simulink subsystem "pulse_logic"  (R2021a)
settings: Solver=VariableStepAuto  StartTime=0.0  StopTime=10.0  RelTol=1e-3
libraries: xbsIndex_r4 x101
settings Model: Creator=casper  LastModifiedBy=casper

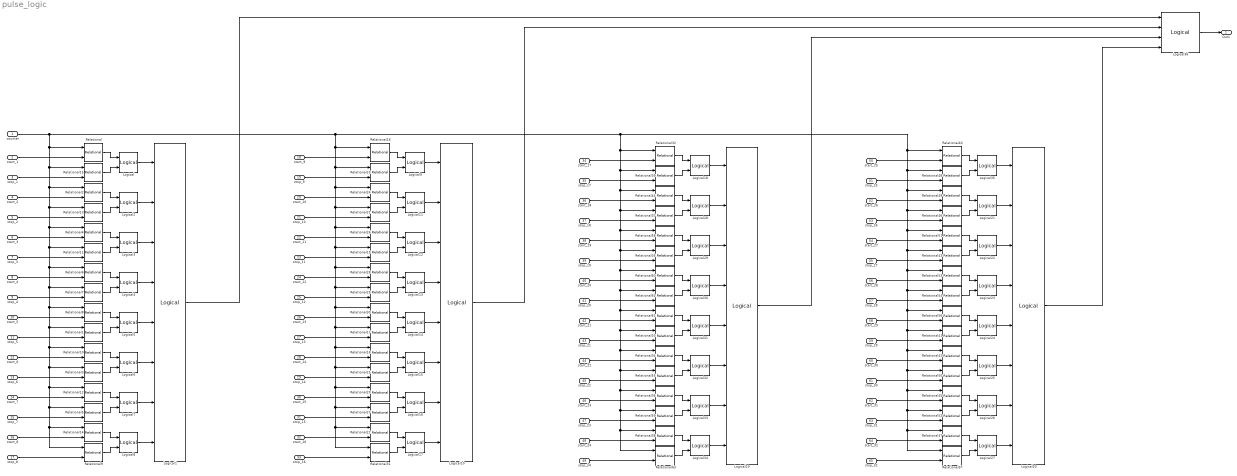
== system pulse_logic ==
  counter : Inport
  start_1 : Inport  Port=2
  stop_1 : Inport  Port=3
  start_2 : Inport  Port=4
  stop_2 : Inport  Port=5
  start_3 : Inport  Port=6
  stop_3 : Inport  Port=7
  start_4 : Inport  Port=8
  stop_4 : Inport  Port=9
  start_5 : Inport  Port=10
  stop_5 : Inport  Port=11
  start_6 : Inport  Port=12
  stop_6 : Inport  Port=13
  start_7 : Inport  Port=14
  stop_7 : Inport  Port=15
  start_8 : Inport  Port=16
  stop_8 : Inport  Port=17
  start_9 : Inport  Port=18
  stop_9 : Inport  Port=19
  start_10 : Inport  Port=20
  stop_10 : Inport  Port=21
  start_11 : Inport  Port=22
  stop_11 : Inport  Port=23
  start_12 : Inport  Port=24
  stop_12 : Inport  Port=25
  start_13 : Inport  Port=26
  stop_13 : Inport  Port=27
  start_14 : Inport  Port=28
  stop_14 : Inport  Port=29
  start_15 : Inport  Port=30
  stop_15 : Inport  Port=31
  start_16 : Inport  Port=32
  stop_16 : Inport  Port=33
  start_17 : Inport  Port=34
  stop_17 : Inport  Port=35
  start_18 : Inport  Port=36
  stop_18 : Inport  Port=37
  start_19 : Inport  Port=38
  stop_19 : Inport  Port=39
  start_20 : Inport  Port=40
  stop_20 : Inport  Port=41
  start_21 : Inport  Port=42
  stop_21 : Inport  Port=43
  start_22 : Inport  Port=44
  stop_22 : Inport  Port=45
  start_23 : Inport  Port=46
  stop_23 : Inport  Port=47
  start_24 : Inport  Port=48
  stop_24 : Inport  Port=49
  start_25 : Inport  Port=50
  stop_25 : Inport  Port=51
  start_26 : Inport  Port=52
  stop_26 : Inport  Port=53
  start_27 : Inport  Port=54
  stop_27 : Inport  Port=55
  start_28 : Inport  Port=56
  stop_28 : Inport  Port=57
  start_29 : Inport  Port=58
  stop_29 : Inport  Port=59
  start_30 : Inport  Port=60
  stop_30 : Inport  Port=61
  start_31 : Inport  Port=62
  stop_31 : Inport  Port=63
  start_32 : Inport  Port=64
  stop_32 : Inport  Port=65
  Logical{,2..9,11..18,21..35} (32 alike) : xbsIndex_r4/Logical  logical_function=AND  inputs=2  en=off  latency=1  precision=Full  arith_type=Unsigned  n_bits=16  bin_pt=0  align_bp=on  dbl_ovrd=off  block_type=logical
  Logical{1,10,19..20} (4 alike) : xbsIndex_r4/Logical  logical_function=OR  inputs=8  en=off  latency=1  precision=Full  arith_type=Unsigned  n_bits=16  bin_pt=0  align_bp=on  dbl_ovrd=off  block_type=logical
  Logical36 : xbsIndex_r4/Logical  logical_function=OR  inputs=4  en=off  latency=1  precision=Full  arith_type=Unsigned  n_bits=16  bin_pt=0  align_bp=on  dbl_ovrd=off  block_type=logical
  Relational{,2,4,6,8,10,12,14,16,18,20,22,24,26,28,30,32,34,36,38,40,42,44..45,47,49,51,53,56,58,60,62} (32 alike) : xbsIndex_r4/Relational  mode=a>=b  op_type=Bool  en=off  latency=1  dbl_ovrd=off  block_type=relational
  Relational{1,3,5,7,9,11,13,15,17,19,21,23,25,27,29,31,33,35,37,39,41,43,46,48,50,52,54..55,57,59,61,63} (32 alike) : xbsIndex_r4/Relational  mode=a<b  op_type=Bool  en=off  latency=1  dbl_ovrd=off  block_type=relational
  Out1 : Outport
  wires:
  Logical5/1 -> Logical1/5
  Relational1/1 -> Logical5/2
  Relational9/1 -> Logical8/2
  Relational8/1 -> Logical5/1
  start_1/1 -> Relational/2
  Logical/1 -> Logical1/1
  stop_8/1 -> Relational9/2
  Relational2/1 -> Logical2/1
  Relational7/1 -> Logical4/2
  Relational6/1 -> Logical4/1
  Relational3/1 -> Logical6/2
  Logical4/1 -> Logical1/4
  start_5/1 -> Relational8/2
  Relational15/1 -> Logical/2
  Logical6/1 -> Logical1/6
  stop_6/1 -> Relational3/2
  stop_5/1 -> Relational1/2
  stop_7/1 -> Relational5/2
  Logical2/1 -> Logical1/2
  stop_1/1 -> Relational15/2
  start_4/1 -> Relational6/2
  stop_3/1 -> Relational11/2
  start_6/1 -> Relational10/2
  Relational4/1 -> Logical3/1
  start_3/1 -> Relational4/2
  Relational10/1 -> Logical6/1
  start_2/1 -> Relational2/2
  Relational/1 -> Logical/1
  stop_2/1 -> Relational13/2
  Logical8/1 -> Logical1/8
  Relational5/1 -> Logical7/2
  Relational11/1 -> Logical3/2
  Relational14/1 -> Logical8/1
  start_7/1 -> Relational12/2
  stop_4/1 -> Relational7/2
  start_8/1 -> Relational14/2
  Logical3/1 -> Logical1/3
  Relational12/1 -> Logical7/1
  Logical7/1 -> Logical1/7
  Relational13/1 -> Logical2/2
  Relational29/1 -> Logical13/2
  stop_12/1 -> Relational29/2
  stop_9/1 -> Relational23/2
  start_16/1 -> Relational22/2
  Logical11/1 -> Logical10/2
  stop_14/1 -> Relational25/2
  start_15/1 -> Relational20/2
  Logical15/1 -> Logical10/6
  Logical17/1 -> Logical10/8
  stop_10/1 -> Relational21/2
  Relational16/1 -> Logical9/1
  Relational24/1 -> Logical11/1
  Logical13/1 -> Logical10/4
  Relational25/1 -> Logical15/2
  Relational17/1 -> Logical14/2
  start_11/1 -> Relational26/2
  start_12/1 -> Relational28/2
  Logical12/1 -> Logical10/3
  Relational20/1 -> Logical16/1
  stop_16/1 -> Relational31/2
  Relational22/1 -> Logical17/1
  Relational27/1 -> Logical16/2
  Logical14/1 -> Logical10/5
  Relational26/1 -> Logical12/1
  start_10/1 -> Relational24/2
  Relational30/1 -> Logical14/1
  start_13/1 -> Relational30/2
  Relational28/1 -> Logical13/1
  Relational21/1 -> Logical11/2
  Relational19/1 -> Logical12/2
  stop_15/1 -> Relational27/2
  stop_13/1 -> Relational17/2
  start_14/1 -> Relational18/2
  Logical16/1 -> Logical10/7
  start_9/1 -> Relational16/2
  stop_11/1 -> Relational19/2
  Relational31/1 -> Logical17/2
  Relational23/1 -> Logical9/2
  Relational18/1 -> Logical15/1
  Logical9/1 -> Logical10/1
  stop_27/1 -> Relational43/2
  Logical26/1 -> Logical20/7
  start_30/1 -> Relational42/2
  stop_29/1 -> Relational41/2
  Relational43/1 -> Logical22/2
  Relational54/1 -> Logical23/2
  Relational33/1 -> Logical31/2
  start_26/1 -> Relational49/2
  Relational36/1 -> Logical33/1
  stop_23/1 -> Relational59/2
  stop_32/1 -> Relational57/2
  Relational41/1 -> Logical24/2
  Logical22/1 -> Logical20/3
  start_27/1 -> Relational51/2
  stop_28/1 -> Relational54/2
  start_18/1 -> Relational44/2
  Relational49/1 -> Logical21/1
  stop_30/1 -> Relational50/2
  Relational47/1 -> Logical27/1
  start_32/1 -> Relational47/2
  Relational53/1 -> Logical23/1
  Relational56/1 -> Logical24/1
  Relational51/1 -> Logical22/1
  Relational45/1 -> Logical26/1
  start_31/1 -> Relational45/2
  counter/1 -> Relational2/1, Relational13/1, Relational4/1, Relational11/1, Relational7/1, Relational8/1, Relational1/1, Relational10/1, Relational5/1, Relational14/1, Relational9/1, Relational12/1, Relational3/1, Relational6/1, Relational15/1, Relational/1, Relational24/1, Relational21/1, Relational26/1, Relational19/1, Relational29/1, Relational30/1, Relational17/1, Relational18/1, Relational27/1, Relational22/1, Relational31/1, Relational20/1, Relational25/1, Relational28/1, Relational23/1, Relational16/1, Relational44/1, Relational37/1, Relational58/1, Relational35/1, Relational61/1, Relational62/1, Relational33/1, Relational34/1, Relational59/1, Relational38/1, Relational63/1, Relational36/1, Relational55/1, Relational60/1, Relational39/1, Relational32/1, Relational49/1, Relational46/1, Relational51/1, Relational43/1, Relational54/1, Relational56/1, Relational41/1, Relational42/1, Relational52/1, Relational47/1, Relational57/1, Relational45/1, Relational50/1, Relational53/1, Relational48/1, Relational40/1
  stop_19/1 -> Relational35/2
  stop_25/1 -> Relational48/2
  stop_26/1 -> Relational46/2
  Logical27/1 -> Logical20/8
  Logical23/1 -> Logical20/4
  Logical25/1 -> Logical20/6
  Relational46/1 -> Logical21/2
  Logical33/1 -> Logical19/7
  start_17/1 -> Relational32/2
  start_29/1 -> Relational56/2
  Relational50/1 -> Logical25/2
  Logical29/1 -> Logical19/3
  Logical19/1 -> Logical36/3
  Logical18/1 -> Logical19/1
  Relational40/1 -> Logical35/1
  stop_21/1 -> Relational33/2
  Logical21/1 -> Logical20/2
  Relational48/1 -> Logical35/2
  Logical30/1 -> Logical19/4
  stop_31/1 -> Relational52/2
  Relational62/1 -> Logical31/1
  Relational37/1 -> Logical28/2
  Logical32/1 -> Logical19/6
  Relational32/1 -> Logical18/1
  Relational61/1 -> Logical30/2
  start_28/1 -> Relational53/2
  start_20/1 -> Relational60/2
  start_19/1 -> Relational58/2
  start_25/1 -> Relational40/2
  Logical24/1 -> Logical20/5
  stop_18/1 -> Relational37/2
  Relational57/1 -> Logical27/2
  Relational42/1 -> Logical25/1
  Logical35/1 -> Logical20/1
  start_21/1 -> Relational62/2
  Logical34/1 -> Logical19/8
  start_23/1 -> Relational36/2
  Logical28/1 -> Logical19/2
  Relational55/1 -> Logical32/2
  Relational44/1 -> Logical28/1
  Relational52/1 -> Logical26/2
  stop_22/1 -> Relational55/2
  Relational38/1 -> Logical34/1
  Relational58/1 -> Logical29/1
  stop_17/1 -> Relational39/2
  Relational63/1 -> Logical34/2
  start_22/1 -> Relational34/2
  start_24/1 -> Relational38/2
  Relational35/1 -> Logical29/2
  Logical31/1 -> Logical19/5
  Relational39/1 -> Logical18/2
  Relational34/1 -> Logical32/1
  stop_20/1 -> Relational61/2
  stop_24/1 -> Relational63/2
  Relational59/1 -> Logical33/2
  Relational60/1 -> Logical30/1
  Logical20/1 -> Logical36/4
  Logical10/1 -> Logical36/2
  Logical36/1 -> Out1/1
  Logical1/1 -> Logical36/1
